simulink model "Experiment1"  (R2025b)
settings: Solver=ode4  StartTime=0.0  StopTime=tsim  FixedStep=baseRate  RelTol=1e-6  AbsTol=1e-6
values from neighbouring files (symbols this model uses):
  a1 = 0.1933    [fmincon_solver_v50.m]    (also in fmincon_solver_v51.m; fmincon_solver_v65_ultrafast.m)
  a2 = 0.1933    [fmincon_solver_v50.m]    (also in fmincon_solver_v51.m; fmincon_solver_v65_ultrafast.m)
  a3 = 0.0621    [fmincon_solver_v50.m]    (also in fmincon_solver_v51.m; fmincon_solver_v65_ultrafast.m)
  b0 = 0.2304    [fmincon_solver_v50.m]    (also in fmincon_solver_v51.m; fmincon_solver_v65_ultrafast.m)
  b1 = 0.1117    [fmincon_solver_v50.m]    (also in fmincon_solver_v51.m; fmincon_solver_v65_ultrafast.m)
  b2 = 0.1057    [fmincon_solver_v50.m]    (also in fmincon_solver_v51.m; fmincon_solver_v65_ultrafast.m)
  b3 = 0.0159    [fmincon_solver_v50.m]    (also in fmincon_solver_v51.m; fmincon_solver_v65_ultrafast.m)
  Gamma1_el = 0.12    [Run_Initializer.m]
  Gamma1_sh = 0.005    [Run_Initializer.m]
  Gamma1_wr = 0.025    [Run_Initializer.m]
  Gamma2_el = 5    [Run_Initializer.m]
  Gamma2_sh = 5    [Run_Initializer.m]
  Gamma2_wr = 5    [Run_Initializer.m]
  Gamma3_el = 10    [Run_Initializer.m]
  Gamma3_sh = 40    [Run_Initializer.m]
  Gamma3_wr = 40    [Run_Initializer.m]
  Gamma4_el = 0.039    [Run_Initializer.m]
  Gamma4_sh = 0.015    [Run_Initializer.m]
  Gamma4_wr = 0.029    [Run_Initializer.m]
  Gamma5_el = 800    [Run_Initializer.m]
  Gamma5_sh = 800    [Run_Initializer.m]
  Gamma5_wr = 800    [Run_Initializer.m]
  Gamma6_el = 0.000001    (= 1e-06)    [Run_Initializer.m]
  Gamma6_sh = 0.005    [Run_Initializer.m]
  Gamma6_wr = 0.02    [Run_Initializer.m]
  Kd_elarm = 0.8    [Run_Initializer.m]
  Kd_sharm = 1.0    (= 1)    [Run_Initializer.m]
  Kd_wrarm = 0.6    [Run_Initializer.m]
  Kp_elarm = 1.2    [Run_Initializer.m]
  Kp_sharm = 1.5    [Run_Initializer.m]
  Kp_wrarm = 1.0    (= 1)    [Run_Initializer.m]
  PWMFreq = 5    [Run_Initializer.m]
  Tz_lim_elarm = .1    (= 0.1)    [Run_Initializer.m]
  Tz_lim_sharm = .1    (= 0.1)    [Run_Initializer.m]
  Tz_lim_wrarm = .1    (= 0.1)    [Run_Initializer.m]
undefined symbols (not defined in the file or in its folder): baseRate, dataRate, DiscIntNeverNeededParam, drop_states_ARM, drop_states_BLACK, drop_states_BLUE, drop_states_RED, F_red_X_nominal, F_red_Y_nominal, F_thrusters_BLACK, F_thrusters_BLUE, F_thrusters_RED, home_states_BLACK, home_states_BLUE, home_states_RED, IBLACK, IBLUE, IDIST, IEE, init_states_BLACK, init_states_BLUE, init_states_RED, IPROX, IRED, K_BLACK, K_BLUE, K_RED, Kd_tb, Kd_tblue, Kd_tr, Kd_xb, Kd_xblue, Kd_xr, Kd_yb, Kd_yblue, Kd_yr, Kp_tb, Kp_tblue, Kp_tr, Kp_xb, Kp_xblue, Kp_xr, Kp_yb, Kp_yblue, Kp_yr, mBLACK, mBLUE, mDIST, mEE, mPROX, mRED, Phase0_End, Phase1_End, Phase2_End, Phase3_End, Phase3_SubPhase1_End, Phase3_SubPhase2_End, Phase3_SubPhase3_End, Phase3_SubPhase4_End, Phase4_End ... (+10)
libraries: simulink x30, nvidiaSharedBlocks x19, MainLibrary x6, dspinverses x3, nvidiaIMUSensorslib x1
(part 1 of 8)
settings Model: Creator=SPOT  LastModifiedBy=ryan
settings OptimizationCC: EnhancedBackFolding=on  PassReuseOutputArgsAs=Individual arguments  ZeroExternalMemoryAtStartup=off  ZeroInternalMemoryAtStartup=off  MaxStackSize=200000  OptimizeBlockOrder=speed  DifferentSizesBufferReuse=on  OptimizationCustomize=off  EfficientTunableParamExpr=on
settings DebuggingCC: ParameterTunabilityLossMsg=error
settings HardwareCC: ProdBitPerLong=64.0  ProdLargestAtomicInteger=LongLong  ProdLargestAtomicFloat=Double  ProdLongLongMode=on  ProdHWDeviceType=ARM Compatible->ARM Cortex-A (64-bit)
settings SFSimCC: MATLABDynamicMemAlloc=off
settings RTWCC: SystemTargetFile=ert.tlc  TemplateMakefile=ert_default_tmf  TargetLang=C++  GPUComputeCapability=3.5  Description=Embedded Coder
settings CodeAppCC: ForceParamTrailComments=on  IgnoreCustomStorageClasses=off  OperatorAnnotations=on  SimulinkDataObjDesc=on  SFDataObjDesc=on  InsertBlockDesc=on
settings ERTTargetCC: InlinedParameterPlacement=Hierarchical  ERTCustomFileTemplate=example_file_process.tlc  DynamicArrayContainerType=coder::array  SupportContinuousTime=on  SupportVariableSizeSignals=on
settings SimscapeCC: SimscapeLogDecimation=1  SimscapeLogDataHistory=5000

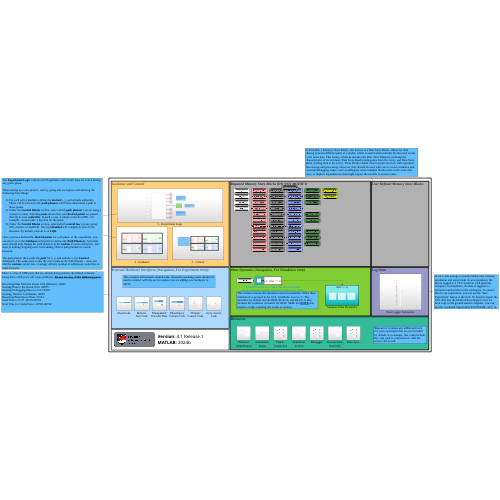
[thumbnail: Simulink's stored preview of the top-level diagram]
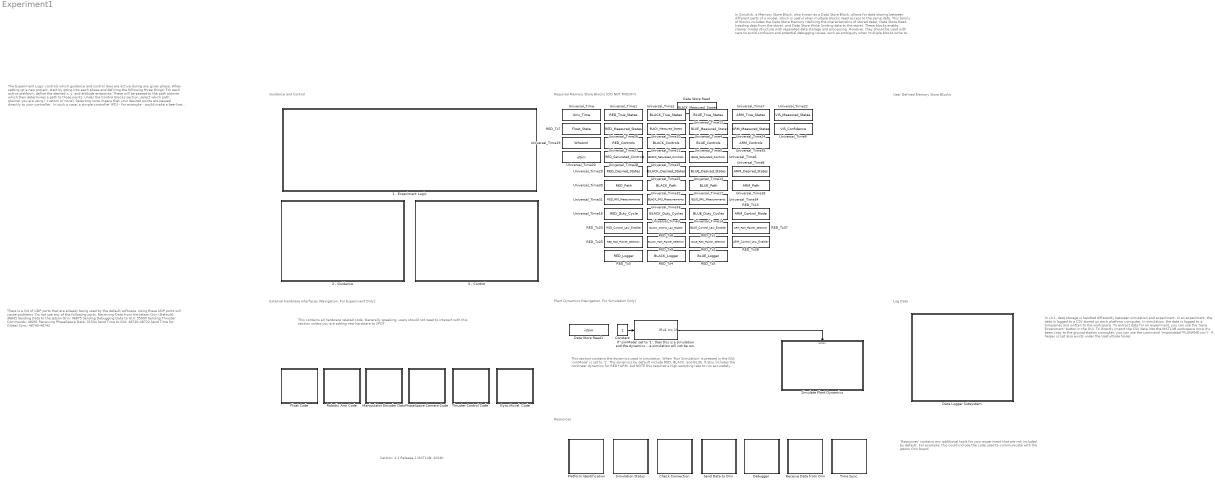
== system Experiment1 ==
  note: Version: 4.1 Release.1
      | MATLAB: 2024b
  note: Required Memory Store Blocks (DO NOT MODIFY)
  note: In Simulink, a Memory Store Block, also known as a Data Store Block, allows for data sharing between different parts of a model, which is useful when multiple blocks need access to the same data. This family of blocks includes the Data Store Memory (defining the characteristics of stored data), Data Store Read (reading data from the store), and Data Store Write (writing data to the store). These blocks enable clearer model structure with separated data storage and processing. However, they should be used with care to avoid confusion and potential debugging issues, such as ambiguity when multiple blocks write to the same data store, or implicit dependencies that might impact the model's execution order.
  note: User Defined Memory Store Blocks
  note: Log Data
  note: In v4.1, data storage is handled differently between simulation and experiment. In an experiment, the data is logged to a CSV stored on each platform computer. In simulation, the data is logged to a timeseries and written to the workspace. To extract data for an experiment, you can use the 'Save Experiment' button in the GUI. To directly import the CSV data into the MATLAB workspace once it's been copy to the ground station computer, you can use the command 'importdata('FILENAME.csv')'. A helper script also exists under the UsefulCode folder.
  note: Resources
  note: 'Resources' contains any additional tools for your experiment that are not included by default. For example, this could include the code used to communicate with the Jetson Orin board.
  note: Plant Dynamics (Navigation, For Simulation Only)
  note: This section contains the dynamics used in simulation. When 'Run Simulation' is pressed in the GUI, 'simMode' is set to '1'. The dynamics by default include RED, BLACK, and BLUE. It also includes the nonlinear dynamics for RED+ARM, but NOTE this requires a high sampling rate to run accurately.
  note: External Hardware Interfaces (Navigation, For Experiment Only):
  note: This contains all hardware related code. Generally speaking, users should not need to interact with this section unless you are adding new hardware to SPOT.
  note: Guidance and Control
  note: The Experiment Logic controls which guidance and control laws are active during any given phase.
      |
      | When setting up a new project, start by going into each phase and defining the following three things:
      |
      | For each active platform, define the desired x, y, and attitude endpoints. These will be passed to the path planner which then determines a path to those points.
      | Under the Control Blocks section, select which path planner you are using ( custom or none). Selecting none means that your desired points are passed directly to your controller . In such a case, a simple controller (PD) - for example - would make a bee-line for the point.
      | Under the Control Blocks section, select which control law you are using (PD, custom, or disabled). Selected disabled will completely turn off the thrusters. By default, custom is an LQR .
      |
      | Once you have defined the desired points for each phase of the experiment, you can move on to the Guidance subsystem to define any Path Planners. Generally, users should only change the path planners in the custom if-action subsytem - but there is nothing stopping users from adding 100s of path planners to switch between.
      |
      | The path planner then sends the path for x, y, and attitude to the Control subsystem. This subsystem works the exact same as the Path Planner - users can edit the custom control law, or simply add any number of additional controllers to jump between.
  note: There is a list of UDP ports that are already being used by the default software. Using these UDP ports will cause problems. Do not use any of the following ports.
      |
      | Receiving Data from the Jetson Orin (Default): 36845
      | Sending Data to the Jetson Orin: 46875
      | Sending Debugging Data to GUI: 55000
      | Sending Thruster Commands: 48291
      | Receiving PhaseSpace Data: 31534
      | Send Time to GUI: 48720-48722
      | Send Time for Global Sync: 48740-48742
  1 - Experiment Logic : Subsystem
  2 - Guidance : Subsystem
  3 - Control : Subsystem
  Check Connection : Subsystem
  Constant : Constant
  Data Logger Subsystem : Subsystem
  Data Store Read : DataStoreRead  DataStoreName=BLACK_Measured_States  IndexOptions=Index vector (dialog)  Indices=1  OutputSizes=1
  Data Store Read1 : DataStoreRead  DataStoreName=isSim  IndexOptions=Index vector (dialog)  Indices=1  OutputSizes=1
  Debugger : Subsystem
  Float Code : Subsystem
  Gyro./Accel. Code : Subsystem
  "If 'simMode' set to '1', then this is a simulation and the dynamics will be simulated. Otherwise, this is an experiment, and the simulation will not be run." : If  IfExpression=u1 == 1  ShowElse=off
  Manipulator Encoder Data : Subsystem
  PhaseSpace Camera Code : Subsystem
  Platform Identification : Subsystem
  RED_Tz1 : DataStoreMemory  DataStoreName=BLUE_Control_Law_Enabler  ReadBeforeWriteMsg=warning  WriteAfterWriteMsg=warning  WriteAfterReadMsg=warning  ShowAdditionalParam=off
  RED_Tz15 : DataStoreMemory  DataStoreName=ARM_Control_Mode  ReadBeforeWriteMsg=warning  WriteAfterWriteMsg=warning  WriteAfterReadMsg=warning  ShowAdditionalParam=off
  RED_Tz2 : DataStoreMemory  DataStoreName=BLUE_Path_Planner_Selection  ReadBeforeWriteMsg=warning  WriteAfterWriteMsg=warning  WriteAfterReadMsg=warning  ShowAdditionalParam=off
  RED_Tz20 : DataStoreMemory  DataStoreName=RED_Control_Law_Enabler  ReadBeforeWriteMsg=warning  WriteAfterWriteMsg=warning  WriteAfterReadMsg=warning  ShowAdditionalParam=off
  RED_Tz25 : DataStoreMemory  DataStoreName=RED_Path_Planner_Selection  ReadBeforeWriteMsg=warning  WriteAfterWriteMsg=warning  WriteAfterReadMsg=warning  ShowAdditionalParam=off
  RED_Tz3 : DataStoreMemory  DataStoreName=RED_Logger  ReadBeforeWriteMsg=warning  WriteAfterWriteMsg=warning  WriteAfterReadMsg=warning  ShowAdditionalParam=off
  RED_Tz37 : DataStoreMemory  DataStoreName=ARM_Path_Planner_Selection  ReadBeforeWriteMsg=warning  WriteAfterWriteMsg=warning  WriteAfterReadMsg=warning  ShowAdditionalParam=off
  RED_Tz38 : DataStoreMemory  DataStoreName=ARM_Control_Law_Enabler  ReadBeforeWriteMsg=warning  WriteAfterWriteMsg=warning  WriteAfterReadMsg=warning  ShowAdditionalParam=off
  RED_Tz4 : DataStoreMemory  DataStoreName=BLACK_Logger  ReadBeforeWriteMsg=warning  WriteAfterWriteMsg=warning  WriteAfterReadMsg=warning  ShowAdditionalParam=off
  RED_Tz5 : DataStoreMemory  DataStoreName=BLUE_Logger  ReadBeforeWriteMsg=warning  WriteAfterWriteMsg=warning  WriteAfterReadMsg=warning  ShowAdditionalParam=off
  RED_Tz7 : DataStoreMemory  DataStoreName=Float_State  ReadBeforeWriteMsg=warning  WriteAfterWriteMsg=warning  WriteAfterReadMsg=warning  ShowAdditionalParam=off
  RED_Tz8 : DataStoreMemory  DataStoreName=BLACK_Control_Law_Enabler  ReadBeforeWriteMsg=warning  WriteAfterWriteMsg=warning  WriteAfterReadMsg=warning  ShowAdditionalParam=off
  RED_Tz9 : DataStoreMemory  DataStoreName=BLACK_Path_Planner_Selection  ReadBeforeWriteMsg=warning  WriteAfterWriteMsg=warning  WriteAfterReadMsg=warning  ShowAdditionalParam=off
  Receive Data from Orin : Subsystem
  Robotic Arm Code : Subsystem
  Send Data to Orin : Subsystem
  Simulate Plant Dynamics : Subsystem  TreatAsAtomicUnit=on
  Simulation Status : Subsystem
  Thruster Control Code : Subsystem  SystemSampleTime=0.1
  Time Sync. : Subsystem
  Universal_Time : DataStoreMemory  DataStoreName=Univ_Time  ReadBeforeWriteMsg=warning  WriteAfterWriteMsg=warning  WriteAfterReadMsg=warning  ShowAdditionalParam=off
  Universal_Time1 : DataStoreMemory  DataStoreName=RED_True_States  ReadBeforeWriteMsg=warning  WriteAfterWriteMsg=warning  WriteAfterReadMsg=warning  InitialValue=[0;0;0;0;0;0;0;0;0]  ShowAdditionalParam=off
  Universal_Time10 : DataStoreMemory  DataStoreName=BLACK_Measured_States  ReadBeforeWriteMsg=warning  WriteAfterWriteMsg=warning  WriteAfterReadMsg=warning  InitialValue=[0;0;0;0;0;0;0;0;0]  ShowAdditionalParam=off
  Universal_Time11 : DataStoreMemory  DataStoreName=BLACK_Controls  ReadBeforeWriteMsg=warning  WriteAfterWriteMsg=warning  WriteAfterReadMsg=warning  InitialValue=[0;0;0]  ShowAdditionalParam=off
  Universal_Time12 : DataStoreMemory  DataStoreName=BLUE_True_States  ReadBeforeWriteMsg=warning  WriteAfterWriteMsg=warning  WriteAfterReadMsg=warning  InitialValue=[0;0;0;0;0;0;0;0;0]  ShowAdditionalParam=off
  Universal_Time13 : DataStoreMemory  DataStoreName=BLUE_Desired_States  ReadBeforeWriteMsg=warning  WriteAfterWriteMsg=warning  WriteAfterReadMsg=warning  InitialValue=[0;0;0]  ShowAdditionalParam=off
  Universal_Time14 : DataStoreMemory  DataStoreName=BLUE_Duty_Cycles  ReadBeforeWriteMsg=warning  WriteAfterWriteMsg=warning  WriteAfterReadMsg=warning  InitialValue=[0;0;0;0;0;0;0;0]  ShowAdditionalParam=off
  Universal_Time15 : DataStoreMemory  DataStoreName=BLACK_Saturated_Controls  ReadBeforeWriteMsg=warning  WriteAfterWriteMsg=warning  WriteAfterReadMsg=warning  InitialValue=[0;0;0]  ShowAdditionalParam=off
  Universal_Time16 : DataStoreMemory  DataStoreName=RED_Duty_Cycle  ReadBeforeWriteMsg=warning  WriteAfterWriteMsg=warning  WriteAfterReadMsg=warning  InitialValue=[0;0;0;0;0;0;0;0]  ShowAdditionalParam=off
  Universal_Time17 : DataStoreMemory  DataStoreName=BLUE_Path  ReadBeforeWriteMsg=warning  WriteAfterWriteMsg=warning  WriteAfterReadMsg=warning  InitialValue=[0;0;0]  ShowAdditionalParam=off
  Universal_Time18 : DataStoreMemory  DataStoreName=ARM_Path  ReadBeforeWriteMsg=warning  WriteAfterWriteMsg=warning  WriteAfterReadMsg=warning  InitialValue=[0;0;0]  ShowAdditionalParam=off
  Universal_Time19 : DataStoreMemory  DataStoreName=WhoAmI  ReadBeforeWriteMsg=warning  WriteAfterWriteMsg=warning  WriteAfterReadMsg=warning  ShowAdditionalParam=off
  Universal_Time2 : DataStoreMemory  DataStoreName=BLACK_True_States  ReadBeforeWriteMsg=warning  WriteAfterWriteMsg=warning  WriteAfterReadMsg=warning  InitialValue=[0;0;0;0;0;0;0;0;0]  ShowAdditionalParam=off
  Universal_Time20 : DataStoreMemory  DataStoreName=isSim  ReadBeforeWriteMsg=warning  WriteAfterWriteMsg=warning  WriteAfterReadMsg=warning  ShowAdditionalParam=off
  Universal_Time22 : DataStoreMemory  DataStoreName=VIS_Measured_States  ReadBeforeWriteMsg=warning  WriteAfterWriteMsg=warning  WriteAfterReadMsg=warning  InitialValue=[0;0;0]  ShowAdditionalParam=off
  Universal_Time24 : DataStoreMemory  DataStoreName=ARM_Measured_States  ReadBeforeWriteMsg=warning  WriteAfterWriteMsg=warning  WriteAfterReadMsg=warning  InitialValue=[0;0;0;0;0;0]  ShowAdditionalParam=off
  Universal_Time25 : DataStoreMemory  DataStoreName=BLACK_Desired_States  ReadBeforeWriteMsg=warning  WriteAfterWriteMsg=warning  WriteAfterReadMsg=warning  InitialValue=[0;0;0]  ShowAdditionalParam=off
  Universal_Time26 : DataStoreMemory  DataStoreName=RED_Measured_States  ReadBeforeWriteMsg=warning  WriteAfterWriteMsg=warning  WriteAfterReadMsg=warning  InitialValue=[0;0;0;0;0;0;0;0;0]  ShowAdditionalParam=off
  Universal_Time27 : DataStoreMemory  DataStoreName=RED_Controls  ReadBeforeWriteMsg=warning  WriteAfterWriteMsg=warning  WriteAfterReadMsg=warning  InitialValue=[0;0;0]  ShowAdditionalParam=off
  Universal_Time28 : DataStoreMemory  DataStoreName=RED_Saturated_Controls  ReadBeforeWriteMsg=warning  WriteAfterWriteMsg=warning  WriteAfterReadMsg=warning  InitialValue=[0;0;0]  ShowAdditionalParam=off
  Universal_Time29 : DataStoreMemory  DataStoreName=RED_Desired_States  ReadBeforeWriteMsg=warning  WriteAfterWriteMsg=warning  WriteAfterReadMsg=warning  InitialValue=[0;0;0]  ShowAdditionalParam=off
  Universal_Time3 : DataStoreMemory  DataStoreName=BLACK_Duty_Cycles  ReadBeforeWriteMsg=warning  WriteAfterWriteMsg=warning  WriteAfterReadMsg=warning  InitialValue=[0;0;0;0;0;0;0;0]  ShowAdditionalParam=off
  Universal_Time30 : DataStoreMemory  DataStoreName=RED_Path  ReadBeforeWriteMsg=warning  WriteAfterWriteMsg=warning  WriteAfterReadMsg=warning  InitialValue=[0;0;0]  ShowAdditionalParam=off
  Universal_Time31 : DataStoreMemory  DataStoreName=RED_IMU_Measurements  ReadBeforeWriteMsg=warning  WriteAfterWriteMsg=warning  WriteAfterReadMsg=warning  InitialValue=[0;0;0]  ShowAdditionalParam=off
  Universal_Time32 : DataStoreMemory  DataStoreName=BLACK_Path  ReadBeforeWriteMsg=warning  WriteAfterWriteMsg=warning  WriteAfterReadMsg=warning  InitialValue=[0;0;0]  ShowAdditionalParam=off
  Universal_Time33 : DataStoreMemory  DataStoreName=BLACK_IMU_Measurements  ReadBeforeWriteMsg=warning  WriteAfterWriteMsg=warning  WriteAfterReadMsg=warning  InitialValue=[0;0;0]  ShowAdditionalParam=off
  Universal_Time34 : DataStoreMemory  DataStoreName=BLUE_IMU_Measurements  ReadBeforeWriteMsg=warning  WriteAfterWriteMsg=warning  WriteAfterReadMsg=warning  InitialValue=[0;0;0]  ShowAdditionalParam=off
  Universal_Time35 : DataStoreMemory  DataStoreName=ARM_Controls  ReadBeforeWriteMsg=warning  WriteAfterWriteMsg=warning  WriteAfterReadMsg=warning  InitialValue=[0;0;0]  ShowAdditionalParam=off
  Universal_Time4 : DataStoreMemory  DataStoreName=BLUE_Measured_States  ReadBeforeWriteMsg=warning  WriteAfterWriteMsg=warning  WriteAfterReadMsg=warning  InitialValue=[0;0;0;0;0;0;0;0;0]  ShowAdditionalParam=off
  Universal_Time5 : DataStoreMemory  DataStoreName=BLUE_Controls  ReadBeforeWriteMsg=warning  WriteAfterWriteMsg=warning  WriteAfterReadMsg=warning  InitialValue=[0;0;0]  ShowAdditionalParam=off
  Universal_Time6 : DataStoreMemory  DataStoreName=BLUE_Saturated_Controls  ReadBeforeWriteMsg=warning  WriteAfterWriteMsg=warning  WriteAfterReadMsg=warning  InitialValue=[0;0;0]  ShowAdditionalParam=off
  Universal_Time7 : DataStoreMemory  DataStoreName=ARM_True_States  ReadBeforeWriteMsg=warning  WriteAfterWriteMsg=warning  WriteAfterReadMsg=warning  InitialValue=[0;0;0;0;0;0]  ShowAdditionalParam=off
  Universal_Time8 : DataStoreMemory  DataStoreName=ARM_Desired_States  ReadBeforeWriteMsg=warning  WriteAfterWriteMsg=warning  WriteAfterReadMsg=warning  InitialValue=[0;0;0]  ShowAdditionalParam=off
  Universal_Time9 : DataStoreMemory  DataStoreName=VIS_Confidence  ReadBeforeWriteMsg=warning  WriteAfterWriteMsg=warning  WriteAfterReadMsg=warning  ShowAdditionalParam=off
  wires:
  "If 'simMode' set to '1', then this is a simulation and the dynamics will be simulated. Otherwise, this is an experiment, and the simulation will not be run."/1 -> Simulate Plant Dynamics/Action
  Constant/1 -> "If 'simMode' set to '1', then this is a simulation and the dynamics will be simulated. Otherwise, this is an experiment, and the simulation will not be run."/1

== system Experiment1/1 - Experiment Logic ==
  note: As a general rule, users should not need to edit these phases. If the initial position must be changed, this change should be made in the GUI.
  note: As a general rule, users should not need to edit these phases. If the home position must be changed, this change should be made in the GUI.
  note: Users should only be editing the sub-systems under Phase #3: Experiment
  Constant : Constant  Value=Phase1_End  SampleTime=-1
  Constant1 : Constant  Value=Phase2_End  SampleTime=-1
  Constant2 : Constant  Value=Phase3_End  SampleTime=-1
  Constant3 : Constant  Value=Phase4_End  SampleTime=-1
  Constant4 : Constant  Value=Phase0_End  SampleTime=-1
  Constant6 : Constant  Value=Phase5_End  SampleTime=-1
  Phase #0: Synchronization : Subsystem  TreatAsAtomicUnit=on
  "Phase #1: Start Floating " : Subsystem  TreatAsAtomicUnit=on
  Phase #2: Initial Position : Subsystem  TreatAsAtomicUnit=on
  Phase #3: Experiment : Subsystem  TreatAsAtomicUnit=on
  Phase #4: Return Home : Subsystem  TreatAsAtomicUnit=on
  Phase #5: Hold Home : Subsystem  TreatAsAtomicUnit=on
  Phase #6: Clean Shutdown : Subsystem  TreatAsAtomicUnit=on
  Separate Phases : If  NumInputs=7  IfExpression=u1 < u2  ElseIfExpressions=(u1 < u3 & u1 >= u2),(u1 < u4 & u1 >= u3), (u1 < u5 & u1 >= u4),(u1 < u6 & u1 >= u5), (u1 < u7 & u1 >= u6) ,(u1 >= u7)  ShowElse=off
  Universal_Time25 : DataStoreRead  DataStoreName=Univ_Time  IndexOptions=Index vector (dialog)  Indices=1  OutputSizes=1
  wires:
  Separate Phases/2 -> "Phase #1: Start Floating "/Action
  Universal_Time25/1 -> Separate Phases/1
  Separate Phases/4 -> Phase #3: Experiment/Action
  Constant2/1 -> Separate Phases/5
  Separate Phases/7 -> Phase #6: Clean Shutdown/Action
  Constant6/1 -> Separate Phases/7
  Separate Phases/6 -> Phase #5: Hold Home/Action
  Separate Phases/1 -> Phase #0: Synchronization/Action
  Constant4/1 -> Separate Phases/2
  Constant/1 -> Separate Phases/3
  Separate Phases/5 -> Phase #4: Return Home/Action
  Separate Phases/3 -> Phase #2: Initial Position/Action
  Constant3/1 -> Separate Phases/6
  Constant1/1 -> Separate Phases/4

== system Experiment1/2 - Guidance ==
  note: Path Planners (RED)
  note: Path Planners (Robotic Manipulator)
  note: Path Planners (BLUE)
  note: Path Planners (BLACK)
  Custom PPL (ARM) : Subsystem  TreatAsAtomicUnit=on
  Custom PPL (BLACK) : Subsystem  TreatAsAtomicUnit=on
  Custom PPL (BLUE) : Subsystem  TreatAsAtomicUnit=on
  Custom PPL (RED) : Subsystem  TreatAsAtomicUnit=on
  Data Store Read : DataStoreRead  DataStoreName=RED_Path_Planner_Selection  IndexOptions=Index vector (dialog)  Indices=1  OutputSizes=1
  Data Store Read1 : DataStoreRead  DataStoreName=BLACK_Path_Planner_Selection  IndexOptions=Index vector (dialog)  Indices=1  OutputSizes=1
  Data Store Read2 : DataStoreRead  DataStoreName=ARM_Path_Planner_Selection  IndexOptions=Index vector (dialog)  Indices=1  OutputSizes=1
  Data Store Read3 : DataStoreRead  DataStoreName=BLUE_Path_Planner_Selection  IndexOptions=Index vector (dialog)  Indices=1  OutputSizes=1
  Data Store Write : DataStoreWrite  DataStoreName=RED_Path  IndexOptions=Index vector (dialog)  Indices=1  OutputSizes=1
  Data Store Write3 : DataStoreWrite  DataStoreName=BLACK_Path  IndexOptions=Index vector (dialog)  Indices=1  OutputSizes=1
  Data Store Write6 : DataStoreWrite  DataStoreName=BLUE_Path  IndexOptions=Index vector (dialog)  Indices=1  OutputSizes=1
  Data Store Write9 : DataStoreWrite  DataStoreName=ARM_Path  IndexOptions=Index vector (dialog)  Indices=1  OutputSizes=1
  Disable PPL (ARM) : Subsystem  TreatAsAtomicUnit=on
  Disable PPL (BLACK) : Subsystem  TreatAsAtomicUnit=on
  Disable PPL (BLUE) : Subsystem  TreatAsAtomicUnit=on
  Disable PPL (RED) : Subsystem  TreatAsAtomicUnit=on
  If : If  IfExpression=u1 == 1
  If1 : If  IfExpression=u1 == 1
  If2 : If  IfExpression=u1 == 2
  If3 : If  IfExpression=u1 == 2
  Merge{,1..3} (4 alike) : Merge
  wires:
  Data Store Read/1 -> If/1
  Merge/1 -> Data Store Write/1
  If/2 -> Disable PPL (RED)/Action
  If/1 -> Custom PPL (RED)/Action
  Disable PPL (RED)/1(Path) -> Merge/2
  Data Store Read1/1 -> If1/1
  Disable PPL (BLACK)/1(Path) -> Merge1/2
  If1/2 -> Disable PPL (BLACK)/Action
  If1/1 -> Custom PPL (BLACK)/Action
  Merge1/1 -> Data Store Write3/1
  Merge2/1 -> Data Store Write6/1
  Disable PPL (BLUE)/1(Path) -> Merge2/2
  If2/2 -> Disable PPL (BLUE)/Action
  If2/1 -> Custom PPL (BLUE)/Action
  Data Store Read3/1 -> If2/1
  If3/1 -> Custom PPL (ARM)/Action
  Merge3/1 -> Data Store Write9/1
  Disable PPL (ARM)/1(Path) -> Merge3/2
  Data Store Read2/1 -> If3/1
  If3/2 -> Disable PPL (ARM)/Action
  Custom PPL (BLUE)/1(Path) -> Merge2/1
  Custom PPL (ARM)/1(Path) -> Merge3/1
  Custom PPL (RED)/1(Path) -> Merge/1
  Custom PPL (BLACK)/1(Path) -> Merge1/1

== system Experiment1/3 - Control ==
  note: Control Laws (RED)
  note: Control Laws (Robotic Manipulator)
  note: Control Laws (BLUE)
  note: Control Laws (BLACK)
  note: The various Control Laws that will be used in any experiment are defined in this subsystem. By Default, a Proportional-Derivative controller is assigned to Control Law #1, and a Linear-Quadratic-Regulator is assigned to Control Law #2.
      |
      | To add new control laws, the recommended approach is to copy is to create a new If Action Subsystem and edit the If block so that it has a new Else-If statement for u1 == 3, u1 ==4, etc. (up to however many controllers you are adding.
      |
      | Then, edit the merge so that it accepts the new number of controllers. Place your new controller into the new If Action subsystem.
      |
      | To use the Control Law, in the Experiment Phases change the input to the relevant Control Law Enabler to match the controller you want to use - in this example, that would be #3.
      |
      | The RED control law section on this page has been configured to have one extra If Action subsystem to demonstrate how this should look when it is properly set up.
      |
      | Note, any controller number that is not assigned (in this case, any number other then 1, 2, and 3) will disable the thrusters due to the Else statement.
  BLACK Controls : DataStoreWrite  DataStoreName=BLACK_Controls  IndexOptions=Index vector (dialog)  Indices=1  OutputSizes=1
  BLUE Controls : DataStoreWrite  DataStoreName=BLUE_Controls  IndexOptions=Index vector (dialog)  Indices=1  OutputSizes=1
  Custom Control (ARM) : Subsystem  TreatAsAtomicUnit=on
  Custom Control (RED) : Subsystem  TreatAsAtomicUnit=on
  Data Store Read1 : DataStoreRead  DataStoreName=RED_Control_Law_Enabler  IndexOptions=Index vector (dialog)  Indices=1  OutputSizes=1
  Data Store Read2 : DataStoreRead  DataStoreName=BLUE_Control_Law_Enabler  IndexOptions=Index vector (dialog)  Indices=1  OutputSizes=1
  Data Store Read3 : DataStoreRead  DataStoreName=BLACK_Control_Law_Enabler  IndexOptions=Index vector (dialog)  Indices=1  OutputSizes=1
  Data Store Read5 : DataStoreRead  DataStoreName=ARM_Control_Law_Enabler  IndexOptions=Index vector (dialog)  Indices=1  OutputSizes=1
  Data Store Write9 : DataStoreWrite  DataStoreName=ARM_Controls  IndexOptions=Index vector (dialog)  Indices=1  OutputSizes=1
  Default LQR Control (BLACK) : Subsystem  TreatAsAtomicUnit=on
  Default LQR Control (BLUE) : Subsystem  TreatAsAtomicUnit=on
  Default LQR Control (RED) : Subsystem  TreatAsAtomicUnit=on
  Default PD (ARM) : Subsystem  TreatAsAtomicUnit=on
  Default PD Control (BLACK) : Subsystem  TreatAsAtomicUnit=on
  Default PD Control (BLUE) : Subsystem  TreatAsAtomicUnit=on
  Default PD Control (RED) : Subsystem  TreatAsAtomicUnit=on
  Disable Control (ARM) : Subsystem  TreatAsAtomicUnit=on
  Disable Thrusters (BLACK) : Subsystem  TreatAsAtomicUnit=on
  Disable Thrusters (BLUE) : Subsystem  TreatAsAtomicUnit=on
  Disable Thrusters (RED) : Subsystem  TreatAsAtomicUnit=on
  If : If  IfExpression=u1 == 1  ElseIfExpressions=u1 == 2, u1 == 3
  If1 : If  IfExpression=u1 == 1  ElseIfExpressions=u1 == 2
  If2 : If  IfExpression=u1 == 1  ElseIfExpressions=u1 == 2
  If3 : If  IfExpression=u1 == 1  ElseIfExpressions=u1 == 2
  Merge : Merge  Inputs=4
  Merge1 : Merge  Inputs=3
  Merge2 : Merge  Inputs=3
  Merge6 : Merge  Inputs=3
  RED Controls : DataStoreWrite  DataStoreName=RED_Controls  IndexOptions=Index vector (dialog)  Indices=1  OutputSizes=1
  wires:
  If/1 -> Default PD Control (RED)/Action
  Data Store Read1/1 -> If/1
  Merge/1 -> RED Controls/1
  If/4 -> Disable Thrusters (RED)/Action
  If/2 -> Default LQR Control (RED)/Action
  If1/1 -> Default PD Control (BLACK)/Action
  If1/2 -> Default LQR Control (BLACK)/Action
  Merge1/1 -> BLACK Controls/1
  Data Store Read3/1 -> If1/1
  If1/3 -> Disable Thrusters (BLACK)/Action
  Data Store Read2/1 -> If2/1
  If2/2 -> Default LQR Control (BLUE)/Action
  If2/3 -> Disable Thrusters (BLUE)/Action
  If2/1 -> Default PD Control (BLUE)/Action
  Merge2/1 -> BLUE Controls/1
  Default PD Control (BLUE)/1(u) -> Merge2/1
  Default LQR Control (BLUE)/1(u) -> Merge2/2
  Disable Thrusters (BLUE)/1(Out1) -> Merge2/3
  Disable Thrusters (BLACK)/1(Out1) -> Merge1/3
  Merge6/1 -> Data Store Write9/1
  If3/3 -> Disable Control (ARM)/Action
  Custom Control (ARM)/1(u) -> Merge6/2
  If3/1 -> Default PD (ARM)/Action
  Disable Control (ARM)/1(Out1) -> Merge6/3
  If3/2 -> Custom Control (ARM)/Action
  Data Store Read5/1 -> If3/1
  Default PD (ARM)/1(u) -> Merge6/1
  Default PD Control (BLACK)/1(u) -> Merge1/1
  Default LQR Control (BLACK)/1(u) -> Merge1/2
  If/3 -> Custom Control (RED)/Action
  Default PD Control (RED)/1(u1) -> Merge/1
  Default LQR Control (RED)/1(u) -> Merge/2
  Custom Control (RED)/1(u) -> Merge/3
  Disable Thrusters (RED)/1(u) -> Merge/4

== system Experiment1/Check Connection ==
  Change BLACK Behavior : Subsystem  TreatAsAtomicUnit=on
  Change BLUE Behavior : Subsystem  TreatAsAtomicUnit=on
  Change RED Behavior : Subsystem  TreatAsAtomicUnit=on
  Data Store Read : DataStoreRead  DataStoreName=WhoAmI  IndexOptions=Index vector (dialog)  Indices=1  OutputSizes=1
  Data Store Read1 : DataStoreRead  DataStoreName=isSim  IndexOptions=Index vector (dialog)  Indices=1  OutputSizes=1
  This IF block determines whether or not to run the BLACK sim/exp : If  NumInputs=2  IfExpression=u1 == 2 & u2 == 0  ShowElse=off
  This IF block determines whether or not to run the BLUE sim/exp : If  NumInputs=2  IfExpression=u1 == 3 & u2 == 0  ShowElse=off
  "This IF block determines whether or not to run the RED sim/exp " : If  NumInputs=2  IfExpression=u1 == 1 & u2 == 0  ShowElse=off
  wires:
  This IF block determines whether or not to run the BLACK sim/exp/1 -> Change BLACK Behavior/Action
  "This IF block determines whether or not to run the RED sim/exp "/1 -> Change RED Behavior/Action
  Data Store Read/1 -> This IF block determines whether or not to run the BLUE sim/exp/1, This IF block determines whether or not to run the BLACK sim/exp/1, "This IF block determines whether or not to run the RED sim/exp "/1
  This IF block determines whether or not to run the BLUE sim/exp/1 -> Change BLUE Behavior/Action
  Data Store Read1/1 -> This IF block determines whether or not to run the BLACK sim/exp/2, This IF block determines whether or not to run the BLUE sim/exp/2, "This IF block determines whether or not to run the RED sim/exp "/2

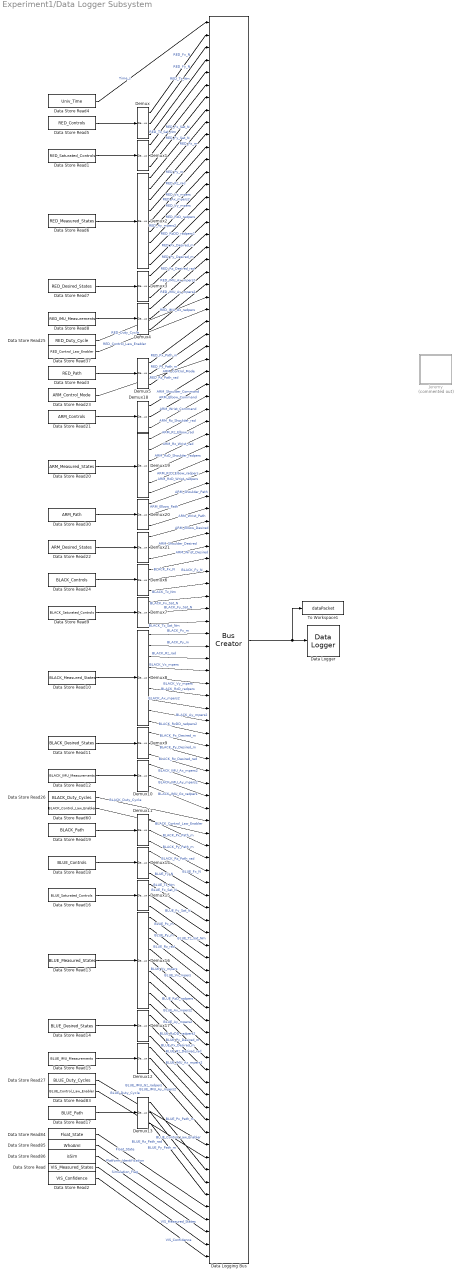
== system Experiment1/Data Logger Subsystem ==
  Data Logger : MainLibrary/Data Logger  SystemSampleTime=-1  VariantActivationTime=update diagram  EmptyChoice=off  PassThrough=off  PassThroughVariantControl=(default)  EmptyChoiceVariantControl=(default)  AllowFlexibleInterface=on  Latency=0  AutoFrameSizeCalculation=off
      settings: SourceProductName=SPOT Custom Library
  Data Logging Bus : BusCreator  Inputs=100
  Data Store Read : DataStoreRead  DataStoreName=VIS_Measured_States  IndexOptions=Index vector (dialog)  Indices=1  OutputSizes=1
  Data Store Read1 : DataStoreRead  DataStoreName=RED_Saturated_Controls  IndexOptions=Index vector (dialog)  Indices=1  OutputSizes=1
  Data Store Read10 : DataStoreRead  DataStoreName=BLACK_Measured_States  IndexOptions=Index vector (dialog)  Indices=1  OutputSizes=1
  Data Store Read11 : DataStoreRead  DataStoreName=BLACK_Desired_States  IndexOptions=Index vector (dialog)  Indices=1  OutputSizes=1
  Data Store Read12 : DataStoreRead  DataStoreName=BLACK_IMU_Measurements  IndexOptions=Index vector (dialog)  Indices=1  OutputSizes=1
  Data Store Read13 : DataStoreRead  DataStoreName=BLUE_Measured_States  IndexOptions=Index vector (dialog)  Indices=1  OutputSizes=1
  Data Store Read14 : DataStoreRead  DataStoreName=BLUE_Desired_States  IndexOptions=Index vector (dialog)  Indices=1  OutputSizes=1
  Data Store Read15 : DataStoreRead  DataStoreName=BLUE_IMU_Measurements  IndexOptions=Index vector (dialog)  Indices=1  OutputSizes=1
  Data Store Read16 : DataStoreRead  DataStoreName=BLUE_Saturated_Controls  IndexOptions=Index vector (dialog)  Indices=1  OutputSizes=1
  Data Store Read17 : DataStoreRead  DataStoreName=BLUE_Path  IndexOptions=Index vector (dialog)  Indices=1  OutputSizes=1
  Data Store Read18 : DataStoreRead  DataStoreName=BLUE_Controls  IndexOptions=Index vector (dialog)  Indices=1  OutputSizes=1
  Data Store Read19 : DataStoreRead  DataStoreName=BLACK_Path  IndexOptions=Index vector (dialog)  Indices=1  OutputSizes=1
  Data Store Read2 : DataStoreRead  DataStoreName=VIS_Confidence  IndexOptions=Index vector (dialog)  Indices=1  OutputSizes=1
  Data Store Read20 : DataStoreRead  DataStoreName=ARM_Measured_States  IndexOptions=Index vector (dialog)  Indices=1  OutputSizes=1
  Data Store Read21 : DataStoreRead  DataStoreName=ARM_Controls  IndexOptions=Index vector (dialog)  Indices=1  OutputSizes=1
  Data Store Read22 : DataStoreRead  DataStoreName=ARM_Desired_States  IndexOptions=Index vector (dialog)  Indices=1  OutputSizes=1
  Data Store Read23 : DataStoreRead  DataStoreName=ARM_Control_Mode  IndexOptions=Index vector (dialog)  Indices=1  OutputSizes=1
  Data Store Read24 : DataStoreRead  DataStoreName=BLACK_Controls  IndexOptions=Index vector (dialog)  Indices=1  OutputSizes=1
  Data Store Read25 : DataStoreRead  DataStoreName=RED_Duty_Cycle  IndexOptions=Index vector (dialog)  Indices=1  OutputSizes=1
  Data Store Read26 : DataStoreRead  DataStoreName=BLACK_Duty_Cycles  IndexOptions=Index vector (dialog)  Indices=1  OutputSizes=1
  Data Store Read27 : DataStoreRead  DataStoreName=BLUE_Duty_Cycles  IndexOptions=Index vector (dialog)  Indices=1  OutputSizes=1
  Data Store Read3 : DataStoreRead  DataStoreName=RED_Path  IndexOptions=Index vector (dialog)  Indices=1  OutputSizes=1
  Data Store Read30 : DataStoreRead  DataStoreName=ARM_Path  IndexOptions=Index vector (dialog)  Indices=1  OutputSizes=1
  Data Store Read37 : DataStoreRead  DataStoreName=RED_Control_Law_Enabler  IndexOptions=Index vector (dialog)  Indices=1  OutputSizes=1
  Data Store Read4 : DataStoreRead  DataStoreName=Univ_Time  IndexOptions=Index vector (dialog)  Indices=1  OutputSizes=1
  Data Store Read5 : DataStoreRead  DataStoreName=RED_Controls  IndexOptions=Index vector (dialog)  Indices=1  OutputSizes=1
  Data Store Read6 : DataStoreRead  DataStoreName=RED_Measured_States  IndexOptions=Index vector (dialog)  Indices=1  OutputSizes=1
  Data Store Read60 : DataStoreRead  DataStoreName=BLACK_Control_Law_Enabler  IndexOptions=Index vector (dialog)  Indices=1  OutputSizes=1
  Data Store Read7 : DataStoreRead  DataStoreName=RED_Desired_States  IndexOptions=Index vector (dialog)  Indices=1  OutputSizes=1
  Data Store Read8 : DataStoreRead  DataStoreName=RED_IMU_Measurements  IndexOptions=Index vector (dialog)  Indices=1  OutputSizes=1
  Data Store Read83 : DataStoreRead  DataStoreName=BLUE_Control_Law_Enabler  IndexOptions=Index vector (dialog)  Indices=1  OutputSizes=1
  Data Store Read84 : DataStoreRead  DataStoreName=Float_State  IndexOptions=Index vector (dialog)  Indices=1  OutputSizes=1
  Data Store Read85 : DataStoreRead  DataStoreName=WhoAmI  IndexOptions=Index vector (dialog)  Indices=1  OutputSizes=1
  Data Store Read86 : DataStoreRead  DataStoreName=isSim  IndexOptions=Index vector (dialog)  Indices=1  OutputSizes=1
  Data Store Read9 : DataStoreRead  DataStoreName=BLACK_Saturated_Controls  IndexOptions=Index vector (dialog)  Indices=1  OutputSizes=1
  Demux{,1,3..7,9..15,17..18,20..21} (18 alike) : Demux  Outputs=3
  Demux16 : Demux  Outputs=9
  Demux19 : Demux  Outputs=6
  Demux2 : Demux  Outputs=9
  Demux8 : Demux  Outputs=9
  Jeremy : Subsystem  Commented=on
  To Workspace1 : ToWorkspace  VariableName=dataPacket  SaveFormat=Timeseries  SampleTime=-1
      settings: Save2DSignal=2-D array (concatenate along first dimension)
  wires:
  Data Store Read/1 -> Data Logging Bus/99  "VIS_Measured_States"
  Data Store Read2/1 -> Data Logging Bus/100  "VIS_Confidence"
  Data Logging Bus/1 -> Data Logger/1, To Workspace1/1
  Demux3/1 -> Data Logging Bus/17  "RED_Px_Desired_m"
  Demux19/1 -> Data Logging Bus/32  "ARM_Rz_Shoulder_rad"
  Demux10/1 -> Data Logging Bus/62  "BLACK_IMU_Ax_mpers2"
  Demux2/1 -> Data Logging Bus/8  "RED_Px_m"
  Demux6/1 -> Data Logging Bus/44  "BLACK_Fx_N"
  Demux16/6 -> Data Logging Bus/81  "BLUE_RzD_radpers"
  Demux8/3 -> Data Logging Bus/52  "BLACK_Rz_rad"
  Data Store Read3/1 -> Demux5/1
  Data Store Read1/1 -> Demux1/1
  Demux8/7 -> Data Logging Bus/56  "BLACK_Ax_mpers2"
  Demux2/9 -> Data Logging Bus/16  "RED_RzDD_radpers2"
  Demux12/2 -> Data Logging Bus/89  "BLUE_IMU_Ay_mpers2"
  Demux2/8 -> Data Logging Bus/15  "RED_Ay_mpers2"
  Demux7/1 -> Data Logging Bus/47  "BLACK_Fx_Sat_N"
  Demux13/3 -> Data Logging Bus/95  "BLUE_Rz_Path_rad"
  Data Store Read16/1 -> Demux15/1
  Demux16/5 -> Data Logging Bus/80  "BLUE_Vy_mpers"
  Demux16/2 -> Data Logging Bus/77  "BLUE_Py_m"
  Data Store Read19/1 -> Demux11/1
  Demux21/2 -> Data Logging Bus/42  "ARM_Shoulder_Desired"
  Data Store Read9/1 -> Demux7/1
  Data Store Read27/1 -> Data Logging Bus/91  "BLUE_Duty_Cycle"
  Demux14/1 -> Data Logging Bus/70  "BLUE_Fx_N"
  Data Store Read8/1 -> Demux4/1
  Demux5/1 -> Data Logging Bus/25  "RED_Px_Path_m"
  Demux21/3 -> Data Logging Bus/43  "ARM_Wrist_Desired"
  Demux16/4 -> Data Logging Bus/79  "BLUE_Vx_mpers"
  Demux5/3 -> Data Logging Bus/27  "RED_Rz_Path_rad"
  Demux8/6 -> Data Logging Bus/55  "BLACK_RzD_radpers"
  Demux16/9 -> Data Logging Bus/84  "BLUE_RzDD_radpers2"
  Data Store Read85/1 -> Data Logging Bus/97  "Platform_Identification"
  Demux18/1 -> Data Logging Bus/29  "ARM_Shoulder_Command"
  Demux16/1 -> Data Logging Bus/76  "BLUE_Px_m"
  Data Store Read17/1 -> Demux13/1
  Demux8/4 -> Data Logging Bus/53  "BLACK_Vx_mpers"
  Demux8/5 -> Data Logging Bus/54  "BLACK_Vy_mpers"
  Demux5/2 -> Data Logging Bus/26  "RED_Py_Path_m"
  Data Store Read21/1 -> Demux18/1
  Demux3/3 -> Data Logging Bus/19  "RED_Rz_Desired_rad"
  Demux6/2 -> Data Logging Bus/45  "BLACK_Fy_N"
  Data Store Read11/1 -> Demux9/1
  Data Store Read12/1 -> Demux10/1
  Data Store Read60/1 -> Data Logging Bus/66  "BLACK_Control_Law_Enabler"
  Data Store Read84/1 -> Data Logging Bus/96  "Float_State"
  Demux17/1 -> Data Logging Bus/85  "BLUE_Px_Desired_m"
  Data Store Read13/1 -> Demux16/1
  Demux6/3 -> Data Logging Bus/46  "BLACK_Tz_Nm"
  Demux11/3 -> Data Logging Bus/69  "BLACK_Rz_Path_rad"
  Demux20/3 -> Data Logging Bus/40  "ARM_Wrist_Path"
  Data Store Read26/1 -> Data Logging Bus/65  "BLACK_Duty_Cycle"
  Demux15/2 -> Data Logging Bus/74  "BLUE_Fy_Sat_N"
  Demux20/2 -> Data Logging Bus/39  "ARM_Elbow_Path"
  Data Store Read22/1 -> Demux21/1
  Data Store Read23/1 -> Data Logging Bus/28  "ARM_Control_Mode"
  Demux2/6 -> Data Logging Bus/13  "RED_RzD_radpers"
  Data Store Read10/1 -> Demux8/1
  Demux9/1 -> Data Logging Bus/59  "BLACK_Px_Desired_m"
  Demux1/1 -> Data Logging Bus/5  "RED_Fx_Sat_N"
  Demux8/8 -> Data Logging Bus/57  "BLACK_Ay_mpers2"
  Data Store Read6/1 -> Demux2/1
  Demux2/7 -> Data Logging Bus/14  "RED_Ax_mpers2"
  Data Store Read5/1 -> Demux/1
  Demux12/3 -> Data Logging Bus/90  "BLUE_IMU_Gz_radpers"
  Demux19/6 -> Data Logging Bus/37  "ARM_RzD_Wrist_radpers"
  Data Store Read18/1 -> Demux14/1
  Demux14/2 -> Data Logging Bus/71  "BLUE_Fy_N"
  Demux10/2 -> Data Logging Bus/63  "BLACK_IMU_Ay_mpers2"
  Demux/1 -> Data Logging Bus/2  "RED_Fx_N"
  Data Store Read30/1 -> Demux20/1
  Demux11/2 -> Data Logging Bus/68  "BLACK_Py_Path_m"
  Demux13/2 -> Data Logging Bus/94  "BLUE_Py_Path_m"
  Data Store Read24/1 -> Demux6/1
  Demux2/5 -> Data Logging Bus/12  "RED_Vy_mpers"
  Demux2/4 -> Data Logging Bus/11  "RED_Vx_mpers"
  Demux14/3 -> Data Logging Bus/72  "BLUE_Tz_Nm"
  Demux16/7 -> Data Logging Bus/82  "BLUE_Ax_mpers2"
  Demux4/1 -> Data Logging Bus/20  "RED_IMU_Ax_mpers2"
  Demux7/2 -> Data Logging Bus/48  "BLACK_Fy_Sat_N"
  Demux4/3 -> Data Logging Bus/22  "RED_IMU_Gz_radpers"
  Demux16/8 -> Data Logging Bus/83  "BLUE_Ay_mpers2"
  Demux8/9 -> Data Logging Bus/58  "BLACK_RzDD_radpers2"
  Data Store Read83/1 -> Data Logging Bus/92  "BLUE_Control_Law_Enabler"
  Demux16/3 -> Data Logging Bus/78  "BLUE_Rz_rad"
  Demux4/2 -> Data Logging Bus/21  "RED_IMU_Ay_mpers2"
  Demux7/3 -> Data Logging Bus/49  "BLACK_Tz_Sat_Nm"
  Demux1/2 -> Data Logging Bus/6  "RED_Fy_Sat_N"
  Demux19/2 -> Data Logging Bus/33  "ARM_Rz_Elbow_rad"
  Demux13/1 -> Data Logging Bus/93  "BLUE_Px_Path_m"
  Data Store Read14/1 -> Demux17/1
  Demux10/3 -> Data Logging Bus/64  "BLACK_IMU_Gz_radpers"
  Data Store Read37/1 -> Data Logging Bus/24  "RED_Control_Law_Enabler"
  Data Store Read86/1 -> Data Logging Bus/98  "Simulation_Flag"
  Demux19/4 -> Data Logging Bus/35  "ARM_RzD_Shoulder_radpers"
  Demux11/1 -> Data Logging Bus/67  "BLACK_Px_Path_m"
  Demux18/2 -> Data Logging Bus/30  "ARM_Elbow_Command"
  Demux15/1 -> Data Logging Bus/73  "BLUE_Fx_Sat_N"
  Demux17/2 -> Data Logging Bus/86  "BLUE_Py_Desired_m"
  Demux19/3 -> Data Logging Bus/34  "ARM_Rz_Wrist_rad"
  Data Store Read15/1 -> Demux12/1
  Demux1/3 -> Data Logging Bus/7  "RED_Tz_Sat_Nm"
  Demux9/3 -> Data Logging Bus/61  "BLACK_Rz_Desired_rad"
  Demux/2 -> Data Logging Bus/3  "RED_Fy_N"
  Demux3/2 -> Data Logging Bus/18  "RED_Py_Desired_m"
  Demux15/3 -> Data Logging Bus/75  "BLUE_Tz_Sat_Nm"
  Demux2/2 -> Data Logging Bus/9  "RED_Py_m"
  Data Store Read7/1 -> Demux3/1
  Demux20/1 -> Data Logging Bus/38  "ARM_Shoulder_Path"
  Data Store Read4/1 -> Data Logging Bus/1  "Time_s"
  Demux2/3 -> Data Logging Bus/10  "RED_Rz_rad"
  Demux8/2 -> Data Logging Bus/51  "BLACK_Py_m"
  Demux8/1 -> Data Logging Bus/50  "BLACK_Px_m"
  Data Store Read20/1 -> Demux19/1
  Demux17/3 -> Data Logging Bus/87  "BLUE_Rz_Desired_rad"
  Demux21/1 -> Data Logging Bus/41  "ARM_Elbow_Desired"
  Data Store Read25/1 -> Data Logging Bus/23  "RED_Duty_Cycle"
  Demux12/1 -> Data Logging Bus/88  "BLUE_IMU_Ax_mpers2"
  Demux19/5 -> Data Logging Bus/36  "ARM_RzD_Elbow_radpers"
  Demux9/2 -> Data Logging Bus/60  "BLACK_Py_Desired_m"
  Demux18/3 -> Data Logging Bus/31  "ARM_Wrist_Command"
  Demux/3 -> Data Logging Bus/4  "RED_Tz_Nm"

== system Experiment1/Debugger ==
  Change BLACK Behavior : Subsystem  TreatAsAtomicUnit=on
  Change BLUE Behavior : Subsystem  TreatAsAtomicUnit=on
  Change RED Behavior : Subsystem  TreatAsAtomicUnit=on
  Data Store Read : DataStoreRead  DataStoreName=WhoAmI  IndexOptions=Index vector (dialog)  Indices=1  OutputSizes=1
  Data Store Read1 : DataStoreRead  DataStoreName=isSim  IndexOptions=Index vector (dialog)  Indices=1  OutputSizes=1
  This IF block determines whether or not to run the BLACK sim/exp : If  NumInputs=2  IfExpression=u1 == 2 & u2 == 0  ShowElse=off
  This IF block determines whether or not to run the BLUE sim/exp : If  NumInputs=2  IfExpression=u1 == 3 & u2 == 0  ShowElse=off
  "This IF block determines whether or not to run the RED sim/exp " : If  NumInputs=2  IfExpression=u1 == 1 & u2 == 0  ShowElse=off
  wires:
  This IF block determines whether or not to run the BLUE sim/exp/1 -> Change BLUE Behavior/Action
  Data Store Read1/1 -> This IF block determines whether or not to run the BLACK sim/exp/2, This IF block determines whether or not to run the BLUE sim/exp/2, "This IF block determines whether or not to run the RED sim/exp "/2
  "This IF block determines whether or not to run the RED sim/exp "/1 -> Change RED Behavior/Action
  Data Store Read/1 -> This IF block determines whether or not to run the BLUE sim/exp/1, This IF block determines whether or not to run the BLACK sim/exp/1, "This IF block determines whether or not to run the RED sim/exp "/1
  This IF block determines whether or not to run the BLACK sim/exp/1 -> Change BLACK Behavior/Action

== system Experiment1/Float Code ==
  note: In this subsection, the "if" statements are used to determine two things: 1) whether or not a simulation is begin performed,
      | then 2) if an experiment is being performed, then which platform is the diagram compiled on. The "IdentifyPlatform" variable
      | is obtained from a text file location on each platform; each text file contains a unique identifier for each platform.
  Data Store Read : DataStoreRead  DataStoreName=isSim  IndexOptions=Index vector (dialog)  Indices=1  OutputSizes=1
  Enable Pucks : Subsystem  TreatAsAtomicUnit=on
  This IF block determines whether or not to run the exp code : If  IfExpression=u1 == 0  ShowElse=off
  wires:
  Data Store Read/1 -> This IF block determines whether or not to run the exp code/1
  This IF block determines whether or not to run the exp code/1 -> Enable Pucks/Action

== system Experiment1/Gyro.//Accel. Code ==
  Data Store Read1 : DataStoreRead  DataStoreName=isSim  IndexOptions=Index vector (dialog)  Indices=1  OutputSizes=1
  Log Gyro/Accel : Subsystem  TreatAsAtomicUnit=on
  This IF block determines whether or not to run the exp code : If  IfExpression=u1 == 0  ShowElse=off
  wires:
  This IF block determines whether or not to run the exp code/1 -> Log Gyro/Accel/Action
  Data Store Read1/1 -> This IF block determines whether or not to run the exp code/1

== system Experiment1/Manipulator Encoder Data ==
  note: This if statement checks if a simulation is being performed. If not, it also checks that this code is being run on the RED platform. If it is, then the arm encoders are used to collect the joint angles. NOTE, the encoder data is collected very slowly, about 0.5 Hz. When the diagram is running faster then this collection rate, previous values of the encoder are held constant.
  Change ARM Behavior : Subsystem  TreatAsAtomicUnit=on
  Data Store Read1 : DataStoreRead  DataStoreName=WhoAmI  IndexOptions=Index vector (dialog)  Indices=1  OutputSizes=1
  Data Store Read2 : DataStoreRead  DataStoreName=isSim  IndexOptions=Index vector (dialog)  Indices=1  OutputSizes=1
  "This IF block determines whether or not to run the RED sim/exp " : If  NumInputs=2  IfExpression=u1 == 1 & u2 == 0  ShowElse=off
  wires:
  Data Store Read2/1 -> "This IF block determines whether or not to run the RED sim/exp "/2
  "This IF block determines whether or not to run the RED sim/exp "/1 -> Change ARM Behavior/Action
  Data Store Read1/1 -> "This IF block determines whether or not to run the RED sim/exp "/1

== system Experiment1/PhaseSpace Camera Code ==
  note: In this subsection, the "if" statement is used to determine if this is a simulation or not. If it is not a simulation, then code is run to receive PhaseSpace camera data via UDP. The PhaseSpace code is currently a standalone executable that should not need to be modified by most users. The code sends all data for all platforms to each platform near simultaneously. If this is a simulation, then no data is required, but a continuous clock is created.
  Data Store Read2 : DataStoreRead  DataStoreName=isSim  IndexOptions=Index vector (dialog)  Indices=1  OutputSizes=1
  "If performing an experiment, grab the PhaseSpace data. Otherwise, use a clock to set time in SIM." : If  IfExpression=u1 == 0  ElseIfExpressions=u1 == 1  ShowElse=off
  Initialize Universal Time (Simulation) : Subsystem  TreatAsAtomicUnit=on
  Use Hardware to Obtain States : Subsystem  TreatAsAtomicUnit=on
  wires:
  Data Store Read2/1 -> "If performing an experiment, grab the PhaseSpace data. Otherwise, use a clock to set time in SIM."/1
  "If performing an experiment, grab the PhaseSpace data. Otherwise, use a clock to set time in SIM."/2 -> Initialize Universal Time (Simulation)/Action
  "If performing an experiment, grab the PhaseSpace data. Otherwise, use a clock to set time in SIM."/1 -> Use Hardware to Obtain States/Action

== system Experiment1/Platform Identification ==
  Data Store Read1 : DataStoreRead  DataStoreName=isSim  IndexOptions=Index vector (dialog)  Indices=1  OutputSizes=1
  "If 'simMode' set to '1', then this is a simulation and the dynamics will be simulated. Otherwise, this is an experiment, and the simulation will not be run." : If  IfExpression=u1 == 0  ShowElse=off
  Subsystem : Subsystem
  wires:
  "If 'simMode' set to '1', then this is a simulation and the dynamics will be simulated. Otherwise, this is an experiment, and the simulation will not be run."/1 -> Subsystem/Action
  Data Store Read1/1 -> "If 'simMode' set to '1', then this is a simulation and the dynamics will be simulated. Otherwise, this is an experiment, and the simulation will not be run."/1

== system Experiment1/Receive Data from Orin ==
  Data Store Read1 : DataStoreRead  DataStoreName=isSim  IndexOptions=Index vector (dialog)  Indices=1  OutputSizes=1
  "If 'simMode' set to '1', then this is a simulation and the dynamics will be simulated. Otherwise, this is an experiment, and the simulation will not be run." : If  IfExpression=u1 == 0  ShowElse=off
  Subsystem : Subsystem
  wires:
  "If 'simMode' set to '1', then this is a simulation and the dynamics will be simulated. Otherwise, this is an experiment, and the simulation will not be run."/1 -> Subsystem/Action
  Data Store Read1/1 -> "If 'simMode' set to '1', then this is a simulation and the dynamics will be simulated. Otherwise, this is an experiment, and the simulation will not be run."/1

== system Experiment1/Robotic Arm Code ==
  note: In this subsection, the "if" statements are used to determine two things: 1) whether or not a simulation is begin performed,
      | then 2) if an experiment is being performed, then which platform is the diagram compiled on. The "IdentifyPlatform" variable
      | is obtained using a custom C++ function which gets the computer name for each platform. NOTE that the arm code only runs on RED.
  Change ARM Behavior : Subsystem  TreatAsAtomicUnit=on
  Data Store Read : DataStoreRead  DataStoreName=WhoAmI  IndexOptions=Index vector (dialog)  Indices=1  OutputSizes=1
  Data Store Read1 : DataStoreRead  DataStoreName=isSim  IndexOptions=Index vector (dialog)  Indices=1  OutputSizes=1
  "This IF block determines whether or not to run the RED sim/exp " : If  NumInputs=2  IfExpression=u1 == 1 & u2 == 0  ShowElse=off
  wires:
  "This IF block determines whether or not to run the RED sim/exp "/1 -> Change ARM Behavior/Action
  Data Store Read1/1 -> "This IF block determines whether or not to run the RED sim/exp "/2
  Data Store Read/1 -> "This IF block determines whether or not to run the RED sim/exp "/1
